simulink model "untitled"  (R2022b)
settings: Solver=VariableStepAuto  StartTime=0.0  StopTime=10.0  RelTol=1e-3
settings Model: Creator=Wikian  LastModifiedBy=Wikian
settings ModelReferenceCC: EnableRefExpFcnMdlSchedulingChecks=on

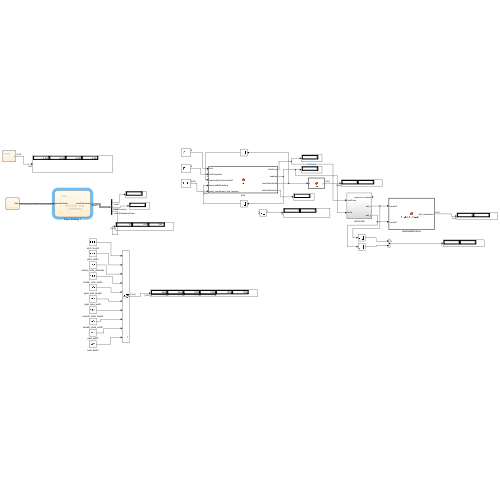
[thumbnail: Simulink's stored preview of the top-level diagram]
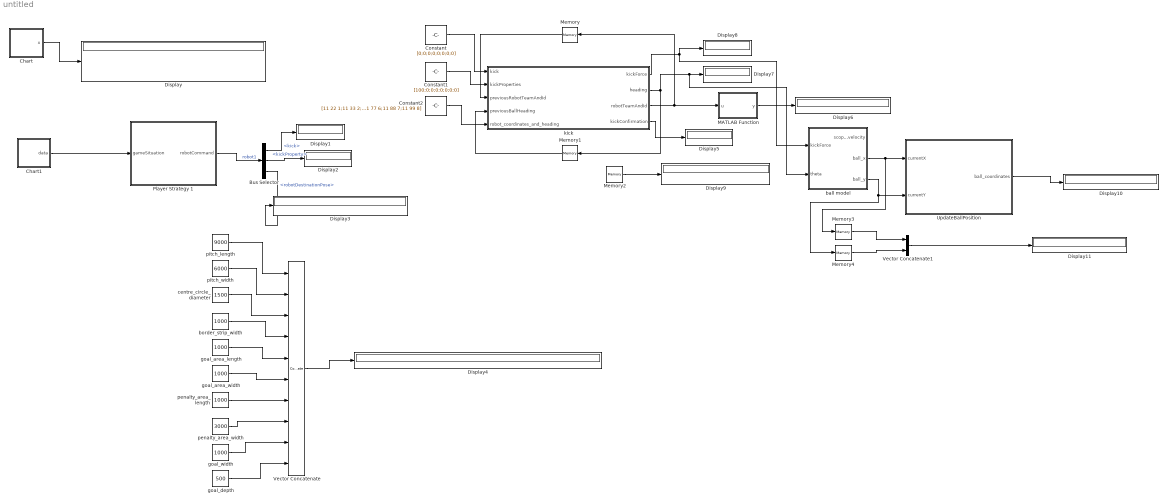
== system untitled ==
  Bus Selector : BusSelector  OutputSignals=kick,kickProperty,robotDestinationPose
  Chart : Stateflow chart  TreatAsAtomicUnit=on
  Chart1 : Stateflow chart  TreatAsAtomicUnit=on
  Constant : Constant  Value=[0;0;0;0;0;0;0;0]
  Constant1 : Constant  Value=[100;0;0;0;0;0;0;0]
  Constant2 : Constant  Value=[11 22 1;11 33 2;11 44 3;11 55 4;11 66 5;11 77 6;11 88 7;11 99 8]
  Display{,1..11} (12 alike) : Display
  MATLAB Function : MATLAB Function  TreatAsAtomicUnit=on
  Memory : Memory  InitialCondition=1  InheritSampleTime=on  LinearizeAsDelay=on
  Memory1 : Memory  InheritSampleTime=on  LinearizeAsDelay=on
  Memory2 : Memory  InitialCondition=[1 1]  InheritSampleTime=on  LinearizeAsDelay=on
  Memory3 : Memory
  Memory4 : Memory
  Player Strategy 1 : Stateflow chart  TreatAsAtomicUnit=on
  UpdateBallPosition : MATLAB Function  TreatAsAtomicUnit=on
  Vector Concatenate : Concatenate  NumInputs=10  Mode=Multidimensional array
  Vector Concatenate1 : Concatenate
  ball model : Subsystem
  border_strip_width : Constant  Value=1000
  centre_circle_diameter : Constant  Value=1500
  goal_area_length : Constant  Value=1000
  goal_area_width : Constant  Value=1000
  goal_depth : Constant  Value=500
  goal_width : Constant  Value=1000
  kick : MATLAB Function  TreatAsAtomicUnit=on
  penalty_area_length : Constant  Value=1000
  penalty_area_width : Constant  Value=3000
  pitch_length : Constant  Value=9000
  pitch_width : Constant  Value=6000
  wires:
  Chart/1(x) -> Display/1
  Chart1/1(data) -> Player Strategy 1/1(gameSituation)
  Player Strategy 1/1(robotCommand) -> Bus Selector/1  "robot1"
  Bus Selector/1 -> Display1/1  "<kick>"
  Bus Selector/2 -> Display2/1  "<kickProperty>"
  Bus Selector/3 -> Display3/1  "<robotDestinationPose>"
  pitch_length/1 -> Vector Concatenate/1
  border_strip_width/1 -> Vector Concatenate/4
  goal_width/1 -> Vector Concatenate/9
  Vector Concatenate/1 -> Display4/1
  pitch_width/1 -> Vector Concatenate/2
  goal_area_width/1 -> Vector Concatenate/6
  penalty_area_width/1 -> Vector Concatenate/8
  centre_circle_diameter/1 -> Vector Concatenate/3
  penalty_area_length/1 -> Vector Concatenate/7
  goal_depth/1 -> Vector Concatenate/10
  goal_area_length/1 -> Vector Concatenate/5
  Constant/1 -> kick/1(kick)
  Constant1/1 -> kick/2(kickProperties)
  Constant2/1 -> kick/5(robot_coordinates_and_heading)
  kick/1(kickForce) -> Display8/1, ball model/1(kickForce)
  kick/3(robotTeamAndId) -> Memory/1, MATLAB Function/1(u)
  kick/4(kickConfirmation) -> Display5/1
  kick/2(heading) -> ball model/2(theta), Display7/1, Memory1/1
  Memory/1 -> kick/3(previousRobotTeamAndId)
  Memory1/1 -> kick/4(previousBallHeading)
  Memory2/1 -> Display9/1
  MATLAB Function/1(y) -> Display6/1
  ball model/2(ball_x) -> Memory3/1, UpdateBallPosition/1(currentX)
  ball model/3(ball_y) -> Memory4/1, UpdateBallPosition/2(currentY)
  UpdateBallPosition/1(ball_coordinates) -> Display10/1
  Memory3/1 -> Vector Concatenate1/1
  Vector Concatenate1/1 -> Display11/1
  Memory4/1 -> Vector Concatenate1/2

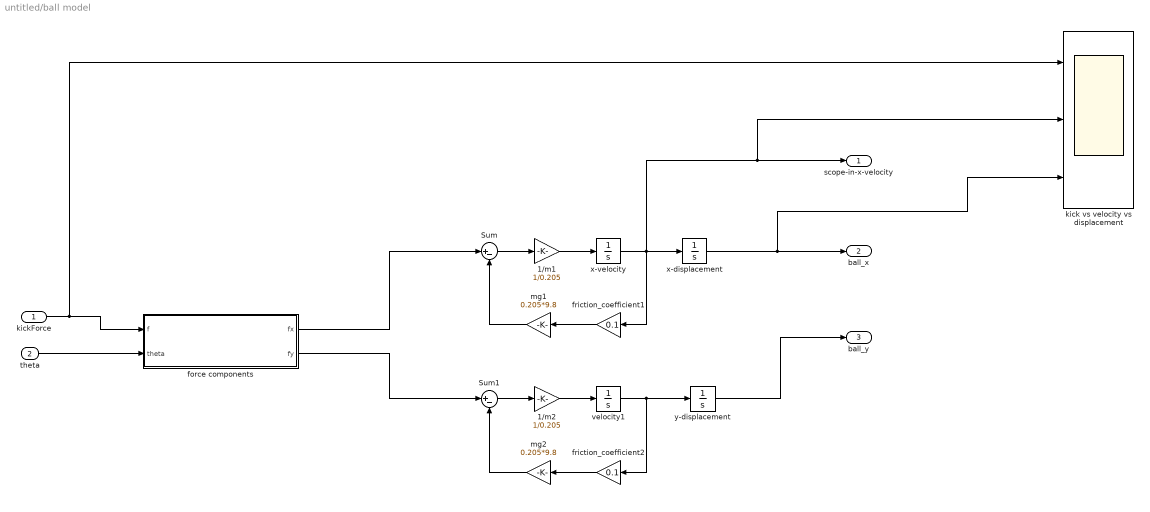
== system untitled/ball model ==
  kickForce : Inport
  theta : Inport  Port=2
  1/m1 : Gain  Gain=1/0.205
  1/m2 : Gain  Gain=1/0.205
  Sum : Sum  Inputs=|+-
  Sum1 : Sum  Inputs=|+-
  force components : MATLAB Function  TreatAsAtomicUnit=on
  friction_coefficient1 : Gain  Gain=0.1
  friction_coefficient2 : Gain  Gain=0.1
  kick vs velocity vs displacement : Scope  NumInputPorts=3
  mg1 : Gain  Gain=0.205*9.8
  mg2 : Gain  Gain=0.205*9.8
  velocity1 : Integrator
  x-displacement : Integrator
  x-velocity : Integrator
  y-displacement : Integrator
  scope-in-x-velocity : Outport
  ball_x : Outport  Port=2
  ball_y : Outport  Port=3
  wires:
  kickForce/1 -> kick vs velocity vs displacement/1, force components/1(f)
  y-displacement/1 -> ball_y/1
  theta/1 -> force components/2(theta)
  x-displacement/1 -> ball_x/1, kick vs velocity vs displacement/3
  mg2/1 -> Sum1/2
  force components/1(fx) -> Sum/1
  1/m1/1 -> x-velocity/1
  Sum1/1 -> 1/m2/1
  force components/2(fy) -> Sum1/1
  friction_coefficient1/1 -> mg1/1
  1/m2/1 -> velocity1/1
  Sum/1 -> 1/m1/1
  mg1/1 -> Sum/2
  friction_coefficient2/1 -> mg2/1
  x-velocity/1 -> x-displacement/1, friction_coefficient1/1, scope-in-x-velocity/1, kick vs velocity vs displacement/2
  velocity1/1 -> y-displacement/1, friction_coefficient2/1

== stateflow chart untitled/Chart1 ==
  state test
    en:
    data.kickConfirmation = false;
    data.ballGameState = 1;
    data.ballCurrentPose = [0 0];
    data.ballLastCommandBy =[1 2];
    data.robotCurrentPose = [1000 1000 0; 2000 2 2;-1000 1000 0;-4000 1000 0 ];
    data.robotCurrentVelocity = [1; 1; 2; 0];
    du:
    ex:
  (default) -> test
  data: data output Bus: gameSituation

== matlab function untitled/MATLAB Function ==
  data: u input; y output
function y = fcn(u)
if u > 4
    y = [2,u-4];
else
    y = [1,u];
end
end

== stateflow chart untitled/Chart ==
  state a
    en:
    a = [1 2 3; 4 5 6; 7 8 9; 10 11 12];
    b = [4 5 6; 7 8 9; 10 11 12; 13 14 15];
    x= [0 0 0 0 ];
    for i=1:1:4
    x(i)=distTo(a(i,1:2),b(i,1:2));
    end
    du:
  (default) -> a
  data: robotPosition function_input; goalPosition function_input; dist function_output; i local; x output; a local =[0 0 0; 0 0 0; 0 0 0; 0 0 0]; b local =[0 0 0; 0 0 0; 0 0 0; 0 0 0]
  function dist = distTo(robotPosition,goalPosition):
    | function dist = distTo(robotPosition,goalPosition)
    |     dist = norm(robotPosition - goalPosition);
    | end

== stateflow chart untitled/Player Strategy 1 ==
  state ROBOT 1 [group]
    (Strategy for robot 1~3)
  state InitialState
    en,du:
    if gameSituation.kickConfirmation == true
    robotCommand.kick = false;
    end
    id = 1; % Team1(Home) Robot 1
    shootDistThres = 2500;
    kickableAreaRadius = 20;
    homeGoalPose = [-5000, 0];
    awayGoalPose = [5000, 0];
    homeAttackPositions = [[2500, 0, 0]; [1500, 2000, 0]; [1500, -2000, 0]; [-2000, 0, 0]];
    homeDefendPositions = [[-1000, 0, 0]; [-3000, 2000, 0]; [-3000, -2000, 0]; [-3500, 0, 0]];
  state Attack
    en,du:
    %%calculate the distance to the goal
    teamDistToGoal = [0 0 0 0];
    for idx=1:1:4
    teamDistToGoal(idx) = distTo(gameSituation.robotCurrentPose(idx,1:2), awayGoalPose);
    end
    distToGoal1 = distTo(gameSituation.robotCurrentPose(id,1:2), awayGoalPose);
    %calculate the distance to the ball
    teamDistToBall = [0 0 0 0];
    for idx=1:1:4
    teamDistToBall(idx) = distTo(gameSituation.robotCurrentPose(idx,1:2), ...
    gameSituation.ballCurrentPose(1:2));
    end
    distToBall = distTo(gameSituation.robotCurrentPose(id,1:2), ...
    gameSituation.ballCurrentPose(1:2))
  state Defend
    en,du:
    %%calculate the distance to the home goal
    teamDistToOwnGoal = [0 0 0 0]
    for idx=1:1:4
    teamDistToOwnGoal(idx) = distTo(gameSituation.robotCurrentPose(idx,1:2), homeGoalPose);
    end
    distToOwnGoal = distTo(gameSituation.robotCurrentPose(id,1:2), homeGoalPose);
  state Position
    en,du:
    playerAttackPosition = homeAttackPositions(id, :);
    kickPower = 1;
    kickState = false;
    desiredPosition = playerAttackPosition;
    isdone = true;
  state Shoot
    en,du:
    angleBallGoal = atan2d(awayGoalPose(2) - gameSituation.ballCurrentPose(2), ...
    awayGoalPose(1) - gameSituation.ballCurrentPose(1));
    kickPower = 100;
    kickState = true;
    kickDirection = 180 + angleBallGoal;
    desiredPosition = [gameSituation.ballCurrentPose(1) + cosd(angleBallGoal) * kickableAreaRadius, ...
    gameSituation.ballCurrentPose(2) + sind(angleBallGoal) * kickableAreaRadius,kickDirection];
    isdone = true;
  state Intercept
    en,du:
    angleBallGoal = atan2d(awayGoalPose(2) - gameSituation.ballCurrentPose(2), ...
    awayGoalPose(1) - gameSituation.ballCurrentPose(1));
    kickPower = 50;
    kickState = true;
    kickDirection = 180 + angleBallGoal;
    desiredPosition = [gameSituation.ballCurrentPose(1) + cosd(angleBallGoal) * kickableAreaRadius, ...
    gameSituation.ballCurrentPose(2) + sind(angleBallGoal) * kickableAreaRadius, kickDirection];
    isdone = true;
  state Formation
    en,du:
    playerDefendPosition = homeDefendPositions(id, :);
    kickPower = 1;
    kickState = false;
    desiredPosition = playerDefendPosition;
    isdone = true;
  state Pass
    en,du:
    [minval,minidx] = min(teamDistToGoal)
    angleBallPlayer = atan2d(gameSituation.robotCurrentPose(minidx, 2) - gameSituation.ballCurrentPose(2), ...
    gameSituation.robotCurrentPose(minidx, 1) - gameSituation.ballCurrentPose(1));
    kickPower = 66;
    kickState = true;
    kickDirection = 180 + angleBallPlayer;
    desiredPosition = [gameSituation.ballCurrentPose(1) + cosd(angleBallPlayer) * kickableAreaRadius, ...
    gameSituation.ballCurrentPose(2) + sind(angleBallPlayer) * kickableAreaRadius, kickDirection];
    isdone = true;
  state Dribble
    en,du:
    angleBallGoal = atan2d(awayGoalPose(2) - gameSituation.ballCurrentPose(2), ...
    awayGoalPose(1) - gameSituation.ballCurrentPose(1));
    kickPower = 33;
    %%should be designed as the kickPower = kickPowerCofficent * 100
    %%kickPowerCofficieant should also be calculated by distance
    kickState = true;
    kickDirection = 180 + angleBallGoal;
    desiredPosition = [gameSituation.ballCurrentPose(1) + cosd(angleBallGoal) * kickableAreaRadius, ...
    gameSituation.ballCurrentPose(2) + sind(angleBallGoal) * kickableAreaRadius, kickDirection];
    isdone = true;
  state Kick
    state MoveTo1
      en,du:
      isdone = false;
      robotCommand.robotDestinationPose = desiredPosition;
    state KickTo
      en,du:
      robotCommand.kick = kickState;
      robotCommand.kickProperty = kickPower;
    MoveTo1 -> KickTo : [gameSituation.robotCurrentPose == robotCommand.robotDestinationPose]
  Position -> MoveTo1 : [isdone]
  Formation -> MoveTo1 : [isdone]
  Intercept -> MoveTo1 : [isdone]
  KickTo -> InitialState : [after(1,sec)]
  Pass -> MoveTo1 : [isdone]
  Shoot -> MoveTo1 : [isdone]
  Dribble -> MoveTo1 : [isdone]
  (default) -> InitialState
  InitialState -> Attack [order 2] : [gameSituation.ballLastCommandBy(1) == 1]
  InitialState -> Defend [order 1] : [gameSituation.ballLastCommandBy(1) == 2]
  Defend -> Intercept [order 1] : [distToOwnGoal ~= max(teamDistToOwnGoal)]
  Defend -> Formation [order 2] : [distToOwnGoal == max(teamDistToOwnGoal)]
  Attack -> Pass [order 3] : [distToGoal1 ~= min(teamDistToGoal)&& distToBall == min(teamDistToBall)]
  Attack -> Dribble [order 4] : [distToBall == min(teamDistToBall) && distToGoal1 == min(teamDistToGoal) && distToGoal1 > shootDistThres]
  Attack -> Shoot [order 2] : [distToBall == min(teamDistToBall) && distToGoal1 == min(teamDistToGoal) && distToGoal1 < shootDistThres]
  Attack -> Position [order 1] : [distToBall ~= min(teamDistToBall)]
  data: robotPosition function_input; goalPosition function_input; dist function_output; awayGoalPose local =[0 0]; homeGoalPose local =[0 0]; id local =1; idx local; angleBallGoal local =0; desiredPosition local =[0 0 0]; distToOwnGoal local =0; kickDirection local =0; kickPower local =0; kickState local =false; minidx local; playerDefendPosition local =[0 0 0]; teamDistToGoal local =[0 0 0 0]; teamDistToOwnGoal local =[0 0 0 0]; minval local; isdone local boolean =false; playerAttackPosition local =[0 0 0]; shootDistThres local =0; gameSituation input Bus: gameSituation; kickableAreaRadius local =0; distToGoal1 local =0; angleBallPlayer local =0; robotCommand output Bus: robotCommand; distToBall local =0; teamDistToBall local =[0 0 0 0]; homeAttackPositions local =[0 0 0;0 0 0;0 0 0;0 0 0]; homeDefendPositions local =[0 0 0;0 0 0;0 0 0;0 0 0]
  function dist = distTo(robotPosition,goalPosition):
    | function dist = distTo(robotPosition,goalPosition)
    |     dist = norm(robotPosition - goalPosition);
    | end

== matlab function untitled/UpdateBallPosition ==
  data: currentX input; ball_coordinates output; currentY input
function ball_coordinates  = UpdateBallPosition(currentX, currentY)

 
    % put heading in vector
    currentPosition = [currentX, currentY];
    
   
    % output the vector
    ball_coordinates = currentPosition;
end

== matlab function untitled/ball model/force components ==
  data: f input; fx output; theta input; fy output
function [fx,fy] = getForceComponents(f, theta)
    
    fx = f*cos((theta*pi)/180);
    fy = f*sin((theta*pi)/180);

end

== matlab function untitled/kick ==
  settings: updateMethod=DISCRETE
  data: kickForce output; heading output; kick input; kickProperties input; robotTeamAndId output; kickConfirmation output; previousRobotTeamAndId input; previousBallHeading input; robot_coordinates_and_heading input
function [kickForce, heading, robotTeamAndId, kickConfirmation] = fcn(kick, kickProperties, previousRobotTeamAndId, previousBallHeading, robot_coordinates_and_heading)

% kick id 8x1 matrix
% has boolean values of whether a robot kicks or not

if all(kick(:) == 0)
    kickForce = 0;
    robotTeamAndId = previousRobotTeamAndId;
    kickConfirmation = false;
    heading = previousBallHeading;

else
    kick_true = find(kick~=0);
    kickingRobotId = kick_true(randi(length(kick_true),1));
    heading = robot_coordinates_and_heading(kickingRobotId,3);
    kickForce = kickProperties(kickingRobotId);
    robotTeamAndId = kickingRobotId;
    kickConfirmation = true;

    
end





end
